simulink model "atelier"  (R2024a)
settings: Solver=VariableStepAuto  StartTime=0.0  StopTime=10.0  RelTol=1e-3
undefined symbols (not defined in the file): g, k, M1, M2, mu, x1_ini, x2_ini
settings Model: Creator=lfgon  LastModifiedBy=lfgon
settings DataIOCC: ReturnWorkspaceOutputs=off

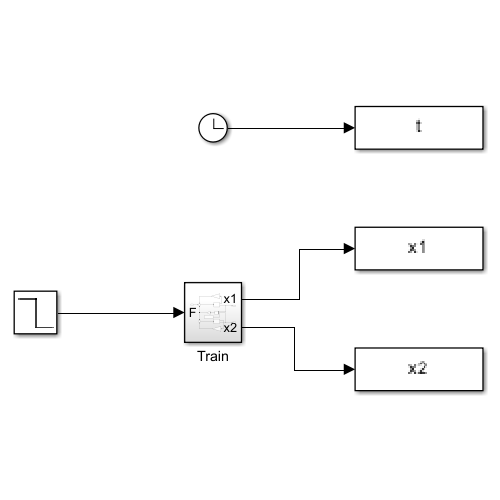
[thumbnail: Simulink's stored preview of the top-level diagram]
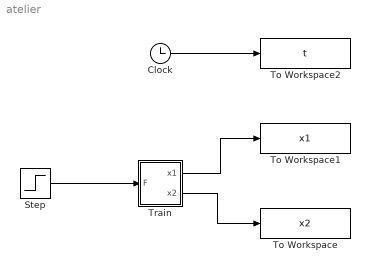
== system atelier ==
  Clock : Clock
  Step : Step  Time=2  Before=0.3  After=0
  To Workspace : ToWorkspace  VariableName=x2  SampleTime=-1
  To Workspace1 : ToWorkspace  VariableName=x1  SampleTime=-1
  To Workspace2 : ToWorkspace  VariableName=t  SampleTime=-1
  Train : Subsystem
  wires:
  Step/1 -> Train/1(F)
  Train/1(x1) -> To Workspace1/1
  Train/2(x2) -> To Workspace/1
  Clock/1 -> To Workspace2/1

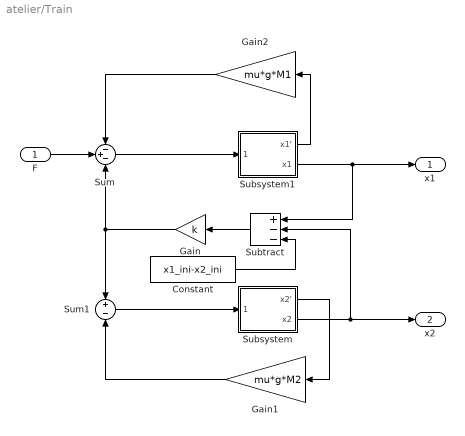
== system atelier/Train ==
  F : Inport
  Constant : Constant  Value=x1_ini-x2_ini
  Gain : Gain  Gain=k
  Gain1 : Gain  Gain=mu*g*M2
  Gain2 : Gain  Gain=mu*g*M1
  Subsystem : Subsystem
  Subsystem1 : Subsystem
  Subtract : Sum  Inputs=+--
  Sum : Sum  Inputs=-+-
  Sum1 : Sum  Inputs=+|-
  x1 : Outport
  x2 : Outport  Port=2
  wires:
  Subsystem1/2(x1) -> x1/1, Subtract/1
  Constant/1 -> Subtract/3
  Sum/1 -> Subsystem1/1(SumF1)
  Subsystem/2(x2) -> x2/1, Subtract/2
  Gain/1 -> Sum/3, Sum1/1
  Subsystem/1(x2') -> Gain1/1
  F/1 -> Sum/2
  Subsystem1/1(x1') -> Gain2/1
  Subtract/1 -> Gain/1
  Gain1/1 -> Sum1/2
  Gain2/1 -> Sum/1
  Sum1/1 -> Subsystem/1(SumF2)

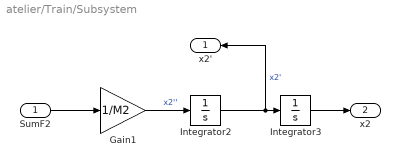
== system atelier/Train/Subsystem ==
  SumF2 : Inport
  Gain1 : Gain  Gain=1/M2
  Integrator2 : Integrator
  Integrator3 : Integrator
  x2' : Outport
  x2 : Outport  Port=2
  wires:
  Integrator2/1 -> x2'/1, Integrator3/1  "x2'"
  Integrator3/1 -> x2/1
  Gain1/1 -> Integrator2/1  "x2''"
  SumF2/1 -> Gain1/1

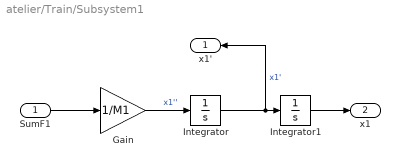
== system atelier/Train/Subsystem1 ==
  SumF1 : Inport
  Gain : Gain  Gain=1/M1
  Integrator : Integrator
  Integrator1 : Integrator
  x1' : Outport
  x1 : Outport  Port=2
  wires:
  SumF1/1 -> Gain/1
  Gain/1 -> Integrator/1  "x1''"
  Integrator1/1 -> x1/1
  Integrator/1 -> x1'/1, Integrator1/1  "x1'"
